simulink model "fb_auto"  (Simulink 10.0)
settings: Solver=ode15s  StartTime=0.0  StopTime=600  RelTol=1e-4  EnableMultiTasking=on
undefined symbols (not defined in the file): sgn, v0
libraries: simulink_need_slupdate x1, simulink x1
settings Model: Creator=prof. G. Celentano  LastModifiedBy=AR
settings DataIOCC: LimitDataPoints=on  SignalLoggingSaveFormat=ModelDataLogs  SignalLoggingName=sigsOut
settings OptimizationCC: ExpressionDepthLimit=2147483647  InitFltsAndDblsToZero=on
settings DebuggingCC: SaveWithParameterizedLinksMsg=none  SignalResolutionControl=TryResolveAllWithWarning  MultiTaskDSMMsg=warning  MultiTaskCondExecSysMsg=none  FcnCallInpInsideContextMsg=warning  StateNameClashWarn=warning
settings HardwareCC: TargetUnknown=on
settings GRTTargetCC: TargetFcnLib=ansi_tfl_tmw.mat

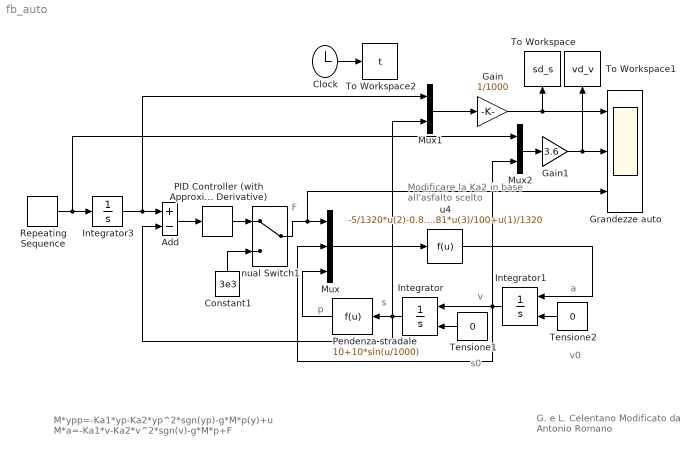
== system fb_auto ==
  note: Modificare la Ka2
      | in base all'asfalto
      | scelto
  note: G. e L. Celentano
      | Modificato da Antonio Romano
  note: v0
  note: s0
  note: F
  note: p
  note: s
  note: v
  note: a
  note: M*ypp=-Ka1*yp-Ka2*yp^2*sgn(yp)-g*M*p(y)+u
      | M*a=-Ka1*v-Ka2*v^2*sgn(v)-g*M*p+F
  Add : Sum  Inputs=+-
  Clock : Clock
  Constant1 : Constant  Value=3e3
  Gain : Gain  Gain=1/1000
  Gain1 : Gain  Gain=3.6
  Grandezze auto : Scope  NumInputPorts=3
  Integrator : Integrator  InitialConditionSource=external  InitialCondition=v0
  Integrator1 : Integrator  InitialConditionSource=external  InitialCondition=v0
  Integrator3 : Integrator
  Mux : Mux  Inputs=3
  Mux1 : Mux  Inputs=2
  Mux2 : Mux  Inputs=2
  PID Controller (with Approximate Derivative) : simulink_need_slupdate/PID Controller (with Approximate Derivative)  P=1320*2*10^2  I=0  D=1320*2*10  N=100
      settings: SourceProductName=Simulink  SourceProductBaseCode=SL
  Pendenza stradale : Fcn  Expr=10+10*sin(u/1000)
  Repeating Sequence : simulink/Sources/Repeating Sequence  rep_seq_t=[0 50 550 600.1]  rep_seq_y=[0 25 25 0]
  Tensione1 : Constant  Value=0
  Tensione2 : Constant  Value=0
  To Workspace : ToWorkspace  VariableName=sd_s  SampleTime=-1
  To Workspace1 : ToWorkspace  VariableName=vd_v  SampleTime=-1
  To Workspace2 : ToWorkspace  VariableName=t  SampleTime=-1
  nual Switch1 : ManualSwitch
  u4 : Fcn  Expr=-5/1320*u(2)-0.80/1320*u(2)^2*sgn(u(2))-9.81*u(3)/100+u(1)/1320
  wires:
  Tensione1/1 -> Integrator/2
  Integrator1/1 -> Integrator/1, Mux/2, Mux2/2
  Tensione2/1 -> Integrator1/2
  u4/1 -> Integrator1/1
  Integrator/1 -> Pendenza stradale/1, Add/2, Mux1/2
  Mux/1 -> u4/1
  Pendenza stradale/1 -> Mux/3
  Add/1 -> PID Controller (with Approximate Derivative)/1
  Gain/1 -> Grandezze auto/1, To Workspace/1
  Mux2/1 -> Gain1/1
  Repeating Sequence/1 -> Integrator3/1, Mux2/1
  Integrator3/1 -> Add/1, Mux1/1
  nual Switch1/1 -> Mux/1, Grandezze auto/3
  Mux1/1 -> Gain/1
  Gain1/1 -> Grandezze auto/2, To Workspace1/1
  Constant1/1 -> nual Switch1/2
  PID Controller (with Approximate Derivative)/1 -> nual Switch1/1
  Clock/1 -> To Workspace2/1
